simulink model "lab1_prbl3"  (R2019a)
settings: Solver=VariableStepAuto  StartTime=0.0  StopTime=120  RelTol=1e-3
settings Model: Creator=criss  LastModifiedBy=criss

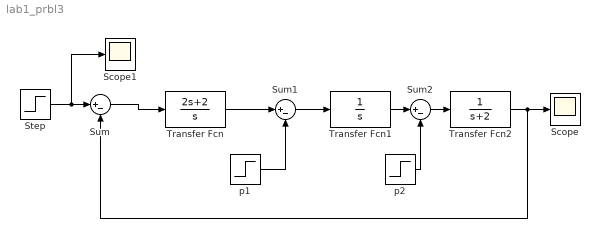
== system lab1_prbl3 ==
  Scope : Scope
  Scope1 : Scope
  Step : Step  Time=0  SampleTime=0
  Sum : Sum  Inputs=|+-
  Sum1 : Sum  Inputs=|+-
  Sum2 : Sum  Inputs=|+-
  Transfer Fcn : TransferFcn  Numerator=[2 2]  Denominator=[1 0]
  Transfer Fcn1 : TransferFcn  Numerator=1  Denominator=[1 0]
  Transfer Fcn2 : TransferFcn  Numerator=1  Denominator=[1 2]
  p1 : Step  Time=30  SampleTime=0
  p2 : Step  Time=60  SampleTime=0
  wires:
  Sum/1 -> Transfer Fcn/1
  Sum2/1 -> Transfer Fcn2/1
  Step/1 -> Scope1/1, Sum/1
  Transfer Fcn1/1 -> Sum2/1
  Sum1/1 -> Transfer Fcn1/1
  Transfer Fcn/1 -> Sum1/1
  p1/1 -> Sum1/2
  p2/1 -> Sum2/2
  Transfer Fcn2/1 -> Sum/2, Scope/1
